simulink model "W04_Town_cs"  (R2019a)
settings: Solver=FixedStepDiscrete  StartTime=0.0  StopTime=15  FixedStep=1/20  RelTol=1e-3
PreLoadFcn:
  | mbxruntime.callbacks.PreLoadFcn(bdroot);
  | check_NUTS_defined
  | model_closed = 0;
  | assignin('base',['model_closed_' bdroot],false);
PostLoadFcn:
  | mbxruntime.callbacks.PostLoadFcn(bdroot);
InitFcn:
  | mbxruntime.callbacks.InitFcn(bdroot);
StartFcn:
  | mbxruntime.callbacks.StartFcn(bdroot);
StopFcn:
  | mbxruntime.callbacks.StopFcn(bdroot);;
  | 
model workspace: external: MAT-File .\W04_Town_cs_hws.mat (data not in the file)
undefined symbols (not defined in the file or in its folder): DiscIntNeverNeededParam, Header, InitImageOutputDir, Poses, Poses_SL_Info, W04_Town_cs_a800676c22972011, W04_Town_cs_bbf210301aa7dfc9, W04_Town_cs_BMW_X5_SUV_1_Dynamics_Empty_STATE_BMW_X5_SUV_1_x0, W04_Town_cs_BMW_X5_SUV_1_Dynamics_Empty_STATE_BMW_X5_SUV_1_y0, W04_Town_cs_BMW_X5_SUV_1_Dynamics_Empty_STATE_BMW_X5_SUV_1_Yaw0, W04_Town_cs_BMW_X5_SUV_1_Dynamics_Empty_STATE_BMW_X5_SUV_1_z0
libraries: adeye_lib x39, PreScanSimulinkLibrary x2, robotlib x2, PreScanUsefulBlocks x1
(part 2 of 3)

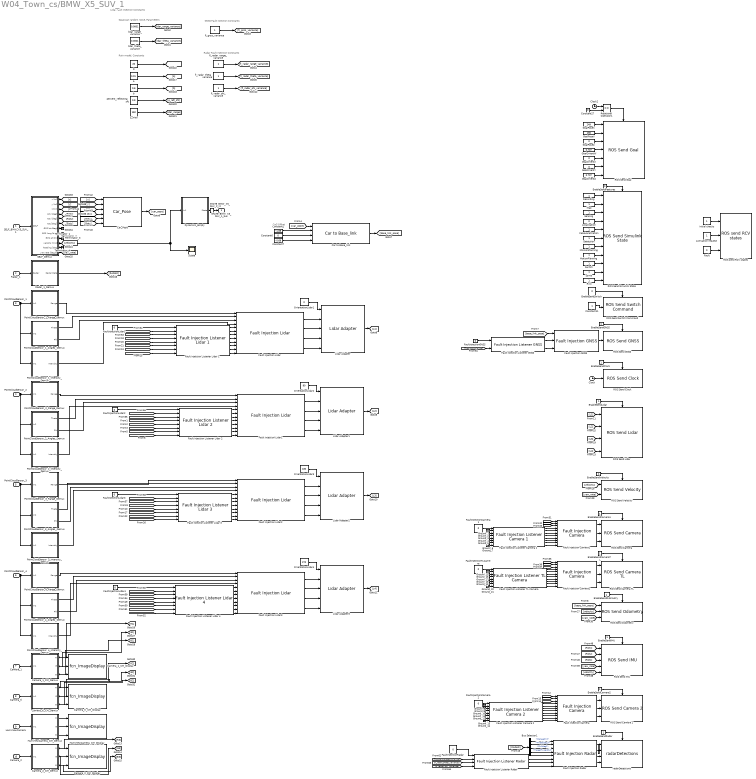
== system W04_Town_cs/BMW_X5_SUV_1 ==
  note: CoG Offset
  note: GNSS Fault Injection Constants
  note: Gaussian random noise, Parameters
  note: Radar Fault Injection Constants
  note: Lidar Fault injection Constants
  note: Rain model, Constants
  SELF_BMW_X5_SUV_1 : Inport  Tag=inport/SelfPort  OutDataTypeStr=Bus: PRESCAN_SELFSENSORDATA  PortDimensions=1  SampleTime=1/20  BusOutputAsStruct=on
  Radar_1 : Inport  Tag=inport/Radar  Port=2  OutDataTypeStr=Bus: PRESCAN_SCANNERSENSOR_MESSAGE  PortDimensions=7  SampleTime=1/20  BusOutputAsStruct=on
  PointCloudSensor_1 : Inport  Tag=inport/PointCloudInport  Port=3  OutDataTypeStr=single  SampleTime=1/20  BusOutputAsStruct=on
  PointCloudSensor_2 : Inport  Tag=inport/PointCloudInport  Port=4  OutDataTypeStr=single  SampleTime=1/20  BusOutputAsStruct=on
  PointCloudSensor_3 : Inport  Tag=inport/PointCloudInport  Port=5  OutDataTypeStr=single  SampleTime=1/20  BusOutputAsStruct=on
  PointCloudSensor_4 : Inport  Tag=inport/PointCloudInport  Port=6  OutDataTypeStr=single  SampleTime=1/20  BusOutputAsStruct=on
  Camera_1 : Inport  Tag=inport/Camera/CameraSensor  Port=7  OutDataTypeStr=uint8  SampleTime=1/20  BusOutputAsStruct=on
  Camera_tl : Inport  Tag=inport/Camera/CameraSensor  Port=8  OutDataTypeStr=uint8  SampleTime=1/20  BusOutputAsStruct=on
  HumViewCamera : Inport  Tag=inport/Camera/CameraSensor  Port=9  OutDataTypeStr=uint8  SampleTime=1/20  BusOutputAsStruct=on
  Camera_2 : Inport  Tag=inport/Camera/CameraSensor  Port=10  OutDataTypeStr=uint8  SampleTime=1/20  BusOutputAsStruct=on
  Activation request : Constant  OutDataTypeStr=Inherit: Inherit via back propagation
  Bus Selector1 : BusSelector  OutputSignals=Range[m],Theta[deg],Phi[deg],TargetTypeID[-]
  Camera_1_CM_Demux : Subsystem  Tag=demux/Camera/Color  mask{SensorName=Camera_1, hres=960, vres=720}
      mask prompts: SensorName "Sensor Name"; hres "Horizontal Resolution"; vres "Vertical Resolution"
      mask Help: eval('openHelp(457)')
      mask Display:
      | fprintf('MONO CAMERA:\n Color\n %s \n %d x %d px',SensorName,hres,vres)
      | port_label('output',1,'R')
      | port_label('output',2,'G')
      | port_label('output',3,'B')
  Camera_1_CM_Display : M-S-Function  Tag=CameraSensor_Color_Display  InitFcn=InitImageOutputDir(gcb);  FunctionName=fcn_ImageDisplay  Parameters=SensorName EnableDisplay EnablePosition DisplayPosition FigureHandle SaveResults BitmapFormat TempOutputDir CameraType DataType  mask(PreScan Color Display Block){SensorName=Camera_1, EnableDisplay=off, EnablePosition=off, DisplayPosition=[10 10 960 720], FigureHandle=1639205, SaveResults=off, Format=PNG, TempOutputDir=0, CameraType=Mono, DataType=uint8}
      mask prompts: SensorName "User Specified: Title of Display"; EnableDisplay "Active"; EnablePosition "Set Display window position"; DisplayPosition "Display window position [xpos ypos width height]"; FigureHandle "Unique Handle"; SaveResults "Save results"; TempOutputDir "OutputDir"; CameraType "Camera Type"; DataType "Image Data Type"
      mask help: This block displays the RGB output of a PreScan camera sensor.
      mask init:
      | if EnableDisplay
      |     EnableString='';
      |     EnableColor='gray';
      | else
      |     EnableString='INACTIVE';
      |     EnableColor='red';
      | end
      | switch Format
      |     case 1
      |         BitmapFormat = 'png';
      |     case 2
      |         BitmapFormat = 'bmp';
      |     case 3
      |         BitmapFormat = 'jpg';
      | end 
      | if CameraType==1
      |     CameraTypeName='MONO';
      |     PortNumber=0;
      | else
      |     CameraTypeName='STEREO';
      |     PortNumber=3;
      | end
      settings: CopyFcn=CopyFcnDisplay  DeleteFcn=PreScanBlockDeleteFcn;  ModelCloseFcn=fcn_ImageDisplay_ModelCloseFcn
      mask Help: eval('openHelp(457)')
      mask Callback EnablePosition:
      | MV=get_param(gcb,'MaskVisibilities');
      | if strcmp(get_param(gcb,'EnablePosition'),'on')
      |     MV{4}='on';
      | else
      |     MV{4}='off';
      | end
      | set_param(gcb,'MaskVisibilities',MV);
      | clear MV;
      mask TypeOptions Format: PNG | BMP | JPG
      mask TypeOptions CameraType: Mono | Stereo
      mask TypeOptions DataType: uint8 | single
      mask Display:
      | color(EnableColor);
      | fprintf('%s\n DISPLAY:\n Color \n %s',EnableString,SensorName)
      | port_label('input',1,'R')
      | port_label('input',2,'G')
      | port_label('input',3,'B')
      | port_label('input',PortNumber+1,'R')
      | port_label('input',PortNumber+2,'G')
      | port_label('input',PortNumber+3,'B')
  Camera_2_CM_Demux : Subsystem  Tag=demux/Camera/Color  mask{SensorName=Camera_2, hres=960, vres=720}
      mask prompts: SensorName "Sensor Name"; hres "Horizontal Resolution"; vres "Vertical Resolution"
      mask Help: eval('openHelp(457)')
      mask Display:
      | fprintf('MONO CAMERA:\n Color\n %s \n %d x %d px',SensorName,hres,vres)
      | port_label('output',1,'R')
      | port_label('output',2,'G')
      | port_label('output',3,'B')
  Camera_2_CM_Display : M-S-Function  Tag=CameraSensor_Color_Display  InitFcn=InitImageOutputDir(gcb);  FunctionName=fcn_ImageDisplay  Parameters=SensorName EnableDisplay EnablePosition DisplayPosition FigureHandle SaveResults BitmapFormat TempOutputDir CameraType DataType  mask(PreScan Color Display Block){SensorName=Camera_2, EnableDisplay=off, EnablePosition=off, DisplayPosition=[10 10 960 720], FigureHandle=1639208, SaveResults=off, Format=PNG, TempOutputDir=0, CameraType=Mono, DataType=uint8}
      mask prompts: SensorName "User Specified: Title of Display"; EnableDisplay "Active"; EnablePosition "Set Display window position"; DisplayPosition "Display window position [xpos ypos width height]"; FigureHandle "Unique Handle"; SaveResults "Save results"; TempOutputDir "OutputDir"; CameraType "Camera Type"; DataType "Image Data Type"
      mask help: This block displays the RGB output of a PreScan camera sensor.
      mask init: same as W04_Town_cs/BMW_X5_SUV_1/Camera_1_CM_Display
      settings: CopyFcn=CopyFcnDisplay  DeleteFcn=PreScanBlockDeleteFcn;  ModelCloseFcn=fcn_ImageDisplay_ModelCloseFcn
      mask Help: eval('openHelp(457)')
      mask Callback EnablePosition:
      | MV=get_param(gcb,'MaskVisibilities');
      | if strcmp(get_param(gcb,'EnablePosition'),'on')
      |     MV{4}='on';
      | else
      |     MV{4}='off';
      | end
      | set_param(gcb,'MaskVisibilities',MV);
      | clear MV;
      mask TypeOptions Format: PNG | BMP | JPG
      mask TypeOptions CameraType: Mono | Stereo
      mask TypeOptions DataType: uint8 | single
      mask Display:
      | color(EnableColor);
      | fprintf('%s\n DISPLAY:\n Color \n %s',EnableString,SensorName)
      | port_label('input',1,'R')
      | port_label('input',2,'G')
      | port_label('input',3,'B')
      | port_label('input',PortNumber+1,'R')
      | port_label('input',PortNumber+2,'G')
      | port_label('input',PortNumber+3,'B')
  Camera_tl_CM_Demux : Subsystem  Tag=demux/Camera/Color  mask{SensorName=Camera_tl, hres=960, vres=720}
      mask prompts: SensorName "Sensor Name"; hres "Horizontal Resolution"; vres "Vertical Resolution"
      mask Help: eval('openHelp(457)')
      mask Display:
      | fprintf('MONO CAMERA:\n Color\n %s \n %d x %d px',SensorName,hres,vres)
      | port_label('output',1,'R')
      | port_label('output',2,'G')
      | port_label('output',3,'B')
  Camera_tl_CM_Display : M-S-Function  Tag=CameraSensor_Color_Display  InitFcn=InitImageOutputDir(gcb);  FunctionName=fcn_ImageDisplay  Parameters=SensorName EnableDisplay EnablePosition DisplayPosition FigureHandle SaveResults BitmapFormat TempOutputDir CameraType DataType  mask(PreScan Color Display Block){SensorName=Camera_tl, EnableDisplay=off, EnablePosition=off, DisplayPosition=[10 10 960 720], FigureHandle=1639206, SaveResults=off, Format=PNG, TempOutputDir=0, CameraType=Mono, DataType=uint8}
      mask prompts: SensorName "User Specified: Title of Display"; EnableDisplay "Active"; EnablePosition "Set Display window position"; DisplayPosition "Display window position [xpos ypos width height]"; FigureHandle "Unique Handle"; SaveResults "Save results"; TempOutputDir "OutputDir"; CameraType "Camera Type"; DataType "Image Data Type"
      mask help: This block displays the RGB output of a PreScan camera sensor.
      mask init: same as W04_Town_cs/BMW_X5_SUV_1/Camera_1_CM_Display
      settings: CopyFcn=CopyFcnDisplay  DeleteFcn=PreScanBlockDeleteFcn;  ModelCloseFcn=fcn_ImageDisplay_ModelCloseFcn
      mask Help: eval('openHelp(457)')
      mask Callback EnablePosition:
      | MV=get_param(gcb,'MaskVisibilities');
      | if strcmp(get_param(gcb,'EnablePosition'),'on')
      |     MV{4}='on';
      | else
      |     MV{4}='off';
      | end
      | set_param(gcb,'MaskVisibilities',MV);
      | clear MV;
      mask TypeOptions Format: PNG | BMP | JPG
      mask TypeOptions CameraType: Mono | Stereo
      mask TypeOptions DataType: uint8 | single
      mask Display:
      | color(EnableColor);
      | fprintf('%s\n DISPLAY:\n Color \n %s',EnableString,SensorName)
      | port_label('input',1,'R')
      | port_label('input',2,'G')
      | port_label('input',3,'B')
      | port_label('input',PortNumber+1,'R')
      | port_label('input',PortNumber+2,'G')
      | port_label('input',PortNumber+3,'B')
  Car to Base_link : adeye_lib/Car to Base_link  SystemSampleTime=-1
  Car_Pose : adeye_lib/Car_Pose  SystemSampleTime=-1
  Clock : Clock
  Clock2 : Clock
  Constant11 : Constant  OutDataTypeStr=Inherit: Inherit via back propagation  SampleTime=0.05
  Constant2 : Constant  Value=-1.69
  Constant27 : Constant  Value=0
  Constant6 : Constant  Value=0
  Constant7 : Constant  Value=-0.69
  Detection : Constant
  Dynamics_Empty : Subsystem  Tag=Dynamics_Empty
      mask Help: eval('openHelp(202)')
      mask Display: port_label('output', 1, 'State');text(0,0,' Empty\n')
  EnableSendCamera1 : Constant  OutDataTypeStr=Inherit: Inherit via back propagation
  EnableSendCamera2 : Constant  OutDataTypeStr=Inherit: Inherit via back propagation
  EnableSendCameraTL : Constant  OutDataTypeStr=Inherit: Inherit via back propagation
  EnableSendClock : Constant  OutDataTypeStr=Inherit: Inherit via back propagation
  EnableSendFeatures : Constant  Value=0  OutDataTypeStr=Inherit: Inherit via back propagation
  EnableSendGNSS : Constant  OutDataTypeStr=Inherit: Inherit via back propagation
  EnableSendIMU : Constant  OutDataTypeStr=Inherit: Inherit via back propagation
  EnableSendLidar : Constant  OutDataTypeStr=Inherit: Inherit via back propagation
  EnableSendOdometry : Constant
  EnableSendRadar : Constant  OutDataTypeStr=Inherit: Inherit via back propagation
  EnableSendSwitch : Constant  Value=0  OutDataTypeStr=Inherit: Inherit via back propagation  SampleTime=0.05
  EnableSendVelocity : Constant  OutDataTypeStr=Inherit: Inherit via back propagation
  FakeLocalization : Constant
  Fault : Constant  Value=0  OutDataTypeStr=Inherit: Inherit via back propagation
  Fault Injection Camera : adeye_lib/Fault Injection Camera  idy=200  idx=100  x=100  y=150  R=0  G=0  B=0
  Fault Injection Camera1 : adeye_lib/Fault Injection Camera  idy=200  idx=100  x=100  y=150  R=0  G=0  B=0
  Fault Injection Camera2 : adeye_lib/Fault Injection Camera  idy=200  idx=100  x=100  y=150  R=0  G=0  B=0
  Fault Injection GNSS : adeye_lib/Fault Injection GNSS  f=20
  Fault Injection Lidar{,1..3} (4 alike) : adeye_lib/Fault Injection Lidar  f=20  p=225*16
  Fault Injection Listener Camera 1 : adeye_lib/Fault Injection Listener Camera 1  SystemSampleTime=-1
  Fault Injection Listener Camera 2 : adeye_lib/Fault Injection Listener Camera 2  SystemSampleTime=-1
  Fault Injection Listener GNSS : adeye_lib/Fault Injection Listener GNSS  SystemSampleTime=-1
  Fault Injection Listener Lidar 1 : adeye_lib/Fault Injection Listener Lidar 1  SystemSampleTime=-1
  Fault Injection Listener Lidar 2 : adeye_lib/Fault Injection Listener Lidar 2  SystemSampleTime=-1
  Fault Injection Listener Lidar 3 : adeye_lib/Fault Injection Listener Lidar 3  SystemSampleTime=-1
  Fault Injection Listener Lidar 4 : adeye_lib/Fault Injection Listener Lidar 4  SystemSampleTime=-1
  Fault Injection Listener Radar : adeye_lib/Fault Injection Listener Radar  SystemSampleTime=-1
  Fault Injection Listener TL Camera : adeye_lib/Fault Injection Listener TL Camera  SystemSampleTime=-1
  Fault Injection Radar : adeye_lib/Fault Injection Radar  n=7
  FaultInjectionCamera1 : Constant  Value=0
  FaultInjectionCamera2 : Constant  Value=0
  FaultInjectionGNSS : Constant  Value=0  OutDataTypeStr=Inherit: Inherit via back propagation  SampleTime=0.05
  FaultInjectionLidar{1..4} (4 alike) : Constant  Value=0  OutDataTypeStr=Inherit: Inherit via back propagation
  FaultInjectionRadar : Constant  Value=0
  FaultInjectionTLCamera : Constant  Value=0
  GoalOrientW : Constant  Value=0.707
  GoalOrientX : Constant  Value=0
  GoalOrientY : Constant  Value=0
  GoalOrientZ : Constant  Value=0.707
  GoalPoseX : Constant  Value=249
  GoalPoseY : Constant  Value=136
  GoalPoseZ : Constant  Value=0
  Ground_{1..21} (21 alike) : Ground
  HumViewCamera_CM_Demux : Subsystem  Tag=demux/Camera/Color  mask{SensorName=HumViewCamera, hres=1871, vres=1080}
      mask prompts: SensorName "Sensor Name"; hres "Horizontal Resolution"; vres "Vertical Resolution"
      mask Help: eval('openHelp(457)')
      mask Display:
      | fprintf('MONO CAMERA:\n Color\n %s \n %d x %d px',SensorName,hres,vres)
      | port_label('output',1,'R')
      | port_label('output',2,'G')
      | port_label('output',3,'B')
  HumViewCamera_CM_Display : M-S-Function  Tag=CameraSensor_Color_Display  InitFcn=InitImageOutputDir(gcb);  FunctionName=fcn_ImageDisplay  Parameters=SensorName EnableDisplay EnablePosition DisplayPosition FigureHandle SaveResults BitmapFormat TempOutputDir CameraType DataType  mask(PreScan Color Display Block){SensorName=HumViewCamera, EnableDisplay=off, EnablePosition=off, DisplayPosition=[10 10 1871 1080], FigureHandle=1639207, SaveResults=off, Format=PNG, TempOutputDir=0, CameraType=Mono, DataType=uint8}
      mask prompts: SensorName "User Specified: Title of Display"; EnableDisplay "Active"; EnablePosition "Set Display window position"; DisplayPosition "Display window position [xpos ypos width height]"; FigureHandle "Unique Handle"; SaveResults "Save results"; TempOutputDir "OutputDir"; CameraType "Camera Type"; DataType "Image Data Type"
      mask help: This block displays the RGB output of a PreScan camera sensor.
      mask init: same as W04_Town_cs/BMW_X5_SUV_1/Camera_1_CM_Display
      settings: CopyFcn=CopyFcnDisplay  DeleteFcn=PreScanBlockDeleteFcn;  ModelCloseFcn=fcn_ImageDisplay_ModelCloseFcn
      mask Help: eval('openHelp(457)')
      mask Callback EnablePosition:
      | MV=get_param(gcb,'MaskVisibilities');
      | if strcmp(get_param(gcb,'EnablePosition'),'on')
      |     MV{4}='on';
      | else
      |     MV{4}='off';
      | end
      | set_param(gcb,'MaskVisibilities',MV);
      | clear MV;
      mask TypeOptions Format: PNG | BMP | JPG
      mask TypeOptions CameraType: Mono | Stereo
      mask TypeOptions DataType: uint8 | single
      mask Display:
      | color(EnableColor);
      | fprintf('%s\n DISPLAY:\n Color \n %s',EnableString,SensorName)
      | port_label('input',1,'R')
      | port_label('input',2,'G')
      | port_label('input',3,'B')
      | port_label('input',PortNumber+1,'R')
      | port_label('input',PortNumber+2,'G')
      | port_label('input',PortNumber+3,'B')
  Initial checks : Constant  OutDataTypeStr=Inherit: Inherit via back propagation
  Lidar Adapter{,1..3} (4 alike) : adeye_lib/Lidar Adapter  SystemSampleTime=-1
  Localization : Constant  Value=0
  Map : Constant
  MissionPlanning : Constant
  MotionPlanning : Constant
  OrientationLidar1 : Constant  Value=0  OutDataTypeStr=Inherit: Inherit via back propagation
  OrientationLidar2 : Constant  Value=90  OutDataTypeStr=Inherit: Inherit via back propagation
  OrientationLidar3 : Constant  Value=180  OutDataTypeStr=Inherit: Inherit via back propagation
  OrientationLidar4 : Constant  Value=270  OutDataTypeStr=Inherit: Inherit via back propagation
  PointCloudSensor_1_Angles_Demux : Subsystem  Tag=demux/PCS/Angles  mask{SensorName=PointCloudSensor_1, offset=225, hres=225, vres=16}
      mask prompts: SensorName "Sensor Name"; offset "Data Start"; hres "Horizontal Resolution"; vres "Vertical Resolution"
      mask Help: eval('openHelp(6400)')
      mask Display:
      | fprintf('Point Cloud:\n Data\n %s \n %d x %d px',SensorName,hres,vres)
      | port_label('output',1,'Theta')
      | port_label('output',2,'Phi')
  PointCloudSensor_1_Intensity_Demux : Subsystem  Tag=demux/PCS/Intensity  mask{SensorName=PointCloudSensor_1, offset=675, hres=225, vres=16}
      mask prompts: SensorName "Sensor Name"; offset "Data Start"; hres "Horizontal Resolution"; vres "Vertical Resolution"
      mask Help: eval('openHelp(6400)')
      mask Display:
      | fprintf('Point Cloud:\n Data\n %s \n %d x %d px',SensorName,hres,vres)
      | port_label('output',1,'Intensity')
  PointCloudSensor_1_Range_Demux : Subsystem  Tag=demux/PCS/Range  mask{SensorName=PointCloudSensor_1, offset=0, hres=225, vres=16}
      mask prompts: SensorName "Sensor Name"; offset "Data Start"; hres "Horizontal Resolution"; vres "Vertical Resolution"
      mask Help: eval('openHelp(6400)')
      mask Display:
      | fprintf('Point Cloud:\n Data\n %s \n %d x %d px',SensorName,hres,vres)
      | port_label('output',1,'Range')
  PointCloudSensor_2_Angles_Demux : Subsystem  Tag=demux/PCS/Angles  mask{SensorName=PointCloudSensor_2, offset=225, hres=225, vres=16}
      mask prompts: SensorName "Sensor Name"; offset "Data Start"; hres "Horizontal Resolution"; vres "Vertical Resolution"
      mask Help: eval('openHelp(6400)')
      mask Display:
      | fprintf('Point Cloud:\n Data\n %s \n %d x %d px',SensorName,hres,vres)
      | port_label('output',1,'Theta')
      | port_label('output',2,'Phi')
  PointCloudSensor_2_Intensity_Demux : Subsystem  Tag=demux/PCS/Intensity  mask{SensorName=PointCloudSensor_2, offset=675, hres=225, vres=16}
      mask prompts: SensorName "Sensor Name"; offset "Data Start"; hres "Horizontal Resolution"; vres "Vertical Resolution"
      mask Help: eval('openHelp(6400)')
      mask Display:
      | fprintf('Point Cloud:\n Data\n %s \n %d x %d px',SensorName,hres,vres)
      | port_label('output',1,'Intensity')
  PointCloudSensor_2_Range_Demux : Subsystem  Tag=demux/PCS/Range  mask{SensorName=PointCloudSensor_2, offset=0, hres=225, vres=16}
      mask prompts: SensorName "Sensor Name"; offset "Data Start"; hres "Horizontal Resolution"; vres "Vertical Resolution"
      mask Help: eval('openHelp(6400)')
      mask Display:
      | fprintf('Point Cloud:\n Data\n %s \n %d x %d px',SensorName,hres,vres)
      | port_label('output',1,'Range')
  PointCloudSensor_3_Angles_Demux : Subsystem  Tag=demux/PCS/Angles  mask{SensorName=PointCloudSensor_3, offset=225, hres=225, vres=16}
      mask prompts: SensorName "Sensor Name"; offset "Data Start"; hres "Horizontal Resolution"; vres "Vertical Resolution"
      mask Help: eval('openHelp(6400)')
      mask Display:
      | fprintf('Point Cloud:\n Data\n %s \n %d x %d px',SensorName,hres,vres)
      | port_label('output',1,'Theta')
      | port_label('output',2,'Phi')
  PointCloudSensor_3_Intensity_Demux : Subsystem  Tag=demux/PCS/Intensity  mask{SensorName=PointCloudSensor_3, offset=675, hres=225, vres=16}
      mask prompts: SensorName "Sensor Name"; offset "Data Start"; hres "Horizontal Resolution"; vres "Vertical Resolution"
      mask Help: eval('openHelp(6400)')
      mask Display:
      | fprintf('Point Cloud:\n Data\n %s \n %d x %d px',SensorName,hres,vres)
      | port_label('output',1,'Intensity')
  PointCloudSensor_3_Range_Demux : Subsystem  Tag=demux/PCS/Range  mask{SensorName=PointCloudSensor_3, offset=0, hres=225, vres=16}
      mask prompts: SensorName "Sensor Name"; offset "Data Start"; hres "Horizontal Resolution"; vres "Vertical Resolution"
      mask Help: eval('openHelp(6400)')
      mask Display:
      | fprintf('Point Cloud:\n Data\n %s \n %d x %d px',SensorName,hres,vres)
      | port_label('output',1,'Range')
  PointCloudSensor_4_Angles_Demux : Subsystem  Tag=demux/PCS/Angles  mask{SensorName=PointCloudSensor_4, offset=225, hres=225, vres=16}
      mask prompts: SensorName "Sensor Name"; offset "Data Start"; hres "Horizontal Resolution"; vres "Vertical Resolution"
      mask Help: eval('openHelp(6400)')
      mask Display:
      | fprintf('Point Cloud:\n Data\n %s \n %d x %d px',SensorName,hres,vres)
      | port_label('output',1,'Theta')
      | port_label('output',2,'Phi')
  PointCloudSensor_4_Intensity_Demux : Subsystem  Tag=demux/PCS/Intensity  mask{SensorName=PointCloudSensor_4, offset=675, hres=225, vres=16}
      mask prompts: SensorName "Sensor Name"; offset "Data Start"; hres "Horizontal Resolution"; vres "Vertical Resolution"
      mask Help: eval('openHelp(6400)')
      mask Display:
      | fprintf('Point Cloud:\n Data\n %s \n %d x %d px',SensorName,hres,vres)
      | port_label('output',1,'Intensity')
  PointCloudSensor_4_Range_Demux : Subsystem  Tag=demux/PCS/Range  mask{SensorName=PointCloudSensor_4, offset=0, hres=225, vres=16}
      mask prompts: SensorName "Sensor Name"; offset "Data Start"; hres "Horizontal Resolution"; vres "Vertical Resolution"
      mask Help: eval('openHelp(6400)')
      mask Display:
      | fprintf('Point Cloud:\n Data\n %s \n %d x %d px',SensorName,hres,vres)
      | port_label('output',1,'Range')
  R : Constant  Value=20
  ROS Send Camera : adeye_lib/ROS Send Camera  SystemSampleTime=-1
  ROS Send Camera 2 : adeye_lib/ROS Send Camera 2  SystemSampleTime=-1
  ROS Send Camera TL : adeye_lib/ROS Send Camera TL  SystemSampleTime=-1
  ROS Send Clock : adeye_lib/ROS Send Clock  SystemSampleTime=-1
  ROS Send GNSS : adeye_lib/ROS Send GNSS  SystemSampleTime=-1
  ROS Send Goal : adeye_lib/ROS Send Goal  SystemSampleTime=-1
  ROS Send IMU : adeye_lib/ROS Send IMU  SystemSampleTime=-1
  ROS Send Lidar : adeye_lib/ROS Send Lidar  SystemSampleTime=-1
  ROS Send Odometry : adeye_lib/ROS Send Odometry  SystemSampleTime=-1
  ROS Send Simulink State : adeye_lib/ROS Send Simulink State  SystemSampleTime=-1
  ROS Send Switch Command : adeye_lib/ROS Send Switch Command  SystemSampleTime=-1
  ROS Send Velocity : adeye_lib/ROS Send Velocity  SystemSampleTime=-1
  ROS send RCV states : adeye_lib/ROS send RCV states  SystemSampleTime=-1
  Radar_1_Demux : Subsystem  Tag=demux/Radar  TreatAsAtomicUnit=on  mask(PreScan Demux Block: Radar){MAXMESSAGES=7}
      mask prompts: MAXMESSAGES "Number of Objects"
      mask help:
      | The Radar Sensor is a detailed sensor based on a physical radar
      | model that includes Antenna GAIN Maps (AGM) and atmospheric
      | attenuation.
      |
      | For more information, please click Help.
      mask Help: eval('openHelp(1464)')
      mask Display:
      | port_label('input',1,'Radar')
      | port_label('output',1,'Radar Data')
  Recording : Constant
  Relational Operator1 : RelationalOperator  Operator===  OutDataTypeStr=boolean  RndMeth=Simplest
  Rviz : Constant
  SELF_Demux : Subsystem  Tag=demux/SelfPort  mask(PreScan Demux Block:){}
      mask help:
      | The SELF port shows (state) information of the actor itself. The outputs are position in the experiment's axis system and the GPS coordinates, and the object's absolute velocity and compass heading.
      |
      | For more information, please click Help.
      settings: DeleteFcn=PreScanBlockDeleteFcn;
      mask Help: eval('openHelp(462)')
      mask Display:
      | port_label('output',1,'x [m]')
      | port_label('output',2,'y [m]')
      | port_label('output',3,'z [m]','texmode','on')
      | port_label('output',4,'Rotx [deg]','texmode','on')
      | port_label('output',5,'Roty [deg]','texmode','on')
      | port_label('output',6,'Rotz [deg]','texmode','on')
      | port_label('output',7,'GPS lat [deg]','texmode','on')
      | port_label('output',8,'GPS long [deg]','texmode','on')
      | port_label('output',9,'GPS alt [m]','texmode','on')
      | port_label('output',10,'Velocity [m/s]')
      | port_label('output',11,'Heading [deg]')
      | port_label('output',12,'Yaw rate [deg/s]')
  STATE_BMW_X5_SUV_1_rc : RateTransition  Tag=mux_rc/StatePort  OutPortSampleTimeOpt=Inherit
  Scope : Scope
  Sensing : Constant
  Ssmp : Constant
  Switch : Constant
  Terminator_{1..4} (4 alike) : Terminator
  a : Constant  Value=0.01
  b : Constant  Value=0.6
  fi_gnss_variance : Constant
  fi_radar_phi_variance : Constant
  fi_radar_range_variance : Constant
  fi_radar_theta_variance : Constant
  lidar_range_variance : Constant  Value=0.0001
  lidar_theta_variance : Constant  Value=0.0001
  percent_reflecting_sfc : Constant  Value=0.9
  radarDetections : adeye_lib/radarDetections  SystemSampleTime=-1
  z_max : Constant  Value=150
  STATE_BMW_X5_SUV_1_bus : Outport  Tag=outport/StatePort  OutDataTypeStr=Bus: PRESCAN_STATEACTUATORDATA  PortDimensions=1  SampleTime=1/20
  wires:
  [x] -> Car_Pose/1
  [y] -> Car_Pose/2
  [z] -> Car_Pose/3
  [Rotx] -> Car_Pose/4
  [Roty] -> Car_Pose/5
  [Rotz] -> Car_Pose/6
  SELF_Demux/12(yaw rate [deg/s]) -> [yaw_rate]
  SELF_Demux/1(x [m]) -> [x]
  SELF_Demux/6(rotz [deg]) -> [Rotz]
  SELF_Demux/5(roty [deg]) -> [Roty]
  SELF_Demux/4(rotx [deg]) -> [Rotx]
  SELF_Demux/3(z [m]) -> [z]
  SELF_Demux/2(y [m]) -> [y]
  Camera_1_CM_Demux/1(R) -> [R1], Camera_1_CM_Display/1
  Camera_1_CM_Demux/2(G) -> [G1], Camera_1_CM_Display/2
  Camera_1_CM_Demux/3(B) -> [B1], Camera_1_CM_Display/3
  Camera_tl_CM_Demux/1(R) -> [R2], Camera_tl_CM_Display/1
  Camera_tl_CM_Demux/2(G) -> [G2], Camera_tl_CM_Display/2
  Camera_tl_CM_Demux/3(B) -> [B2], Camera_tl_CM_Display/3
  Camera_2_CM_Demux/1(R) -> [R3], Camera_2_CM_Display/1
  Camera_2_CM_Demux/2(G) -> [G3], Camera_2_CM_Display/2
  Camera_2_CM_Demux/3(B) -> [B3], Camera_2_CM_Display/3
  Car_Pose/1 -> [car_pose]
  SELF_Demux/10(velocity [m/s]) -> Scope/1, Dynamics_Empty/1(In1), [velocity]
  Radar_1_Demux/1(Radar Data) -> [RADAR]
  [car_pose] -> Car to Base_link/1
  Constant7/1 -> Car to Base_link/4
  Constant6/1 -> Car to Base_link/3
  Car to Base_link/1 -> [base_link_pose]
  Constant2/1 -> Car to Base_link/2
  Fault Injection Camera2/3 -> ROS Send Camera TL/3
  Ssmp/1 -> ROS Send Simulink State/10
  Fault Injection Listener TL Camera/7 -> Fault Injection Camera2/10
  [fi_radar_phi_variance] -> Fault Injection Listener Radar/4
  [G2] -> Fault Injection Camera2/2
  [fi_radar_theta_variance] -> Fault Injection Listener Radar/3
  [fi_radar_range_variance] -> Fault Injection Listener Radar/2
  Fault Injection Listener Camera 2/3 -> Fault Injection Camera/6
  GoalOrientZ/1 -> ROS Send Goal/7
  Fault Injection Listener Camera 1/4 -> Fault Injection Camera1/7
  EnableSendFeatures/1 -> ROS Send Simulink State/Enable
  Fault Injection Listener Radar/4 -> Fault Injection Radar/8
  Fault Injection Listener Radar/3 -> Fault Injection Radar/7
  EnableSendGNSS/1 -> ROS Send GNSS/Enable
  Fault Injection Listener Camera 2/7 -> Fault Injection Camera/10
  Fault Injection Listener Camera 2/4 -> Fault Injection Camera/7
  [yaw_rate] -> ROS Send IMU/4
  Fault/1 -> ROS send RCV states/3
  Fault Injection Listener Camera 2/8 -> Fault Injection Camera/11
  Fault Injection Listener Camera 2/5 -> Fault Injection Camera/8
  Fault Injection Listener Camera 1/7 -> Fault Injection Camera1/10
  Fault Injection Radar/2 -> radarDetections/2
  Fault Injection Listener Camera 1/3 -> Fault Injection Camera1/6
  GoalOrientW/1 -> ROS Send Goal/4
  [G1] -> Fault Injection Camera1/2
  EnableSendSwitch/1 -> ROS Send Switch Command/Enable
  Fault Injection Listener TL Camera/6 -> Fault Injection Camera2/9
  Fault Injection Listener Camera 1/6 -> Fault Injection Camera1/9
  Fault Injection Listener TL Camera/2 -> Fault Injection Camera2/5
  [fi_gnss_variance] -> Fault Injection Listener GNSS/2
  Fault Injection Listener Camera 1/2 -> Fault Injection Camera1/5
  Fault Injection Listener Camera 1/8 -> Fault Injection Camera1/11
  MissionPlanning/1 -> ROS Send Simulink State/7
  Fault Injection Listener TL Camera/5 -> Fault Injection Camera2/8
  Fault Injection Listener TL Camera/3 -> Fault Injection Camera2/6
  Fault Injection Listener TL Camera/4 -> Fault Injection Camera2/7
  Detection/1 -> ROS Send Simulink State/6
  Fault Injection Listener Camera 2/2 -> Fault Injection Camera/5
  GoalOrientX/1 -> ROS Send Goal/5
  Fault Injection Listener Camera 2/6 -> Fault Injection Camera/9
  [L4] -> ROS Send Lidar/4
  GoalOrientY/1 -> ROS Send Goal/6
  EnableSendLidar/1 -> ROS Send Lidar/Enable
  Fault Injection GNSS/1 -> ROS Send GNSS/1
  [velocity] -> ROS Send Odometry/2
  Fault Injection Camera1/3 -> ROS Send Camera/3
  Fault Injection Camera1/2 -> ROS Send Camera/2
  Recording/1 -> ROS Send Simulink State/1
  EnableSendClock/1 -> ROS Send Clock/Enable
  Fault Injection Camera/3 -> ROS Send Camera 2/3
  [L1] -> ROS Send Lidar/1
  Bus Selector1/1 -> Fault Injection Radar/1  "<Range[m]>"
  EnableSendIMU/1 -> ROS Send IMU/Enable
  Fault Injection Listener Camera 1/1 -> Fault Injection Camera1/4
  [base_link_pose] -> Fault Injection GNSS/1
  Fault Injection Listener Camera 2/1 -> Fault Injection Camera/4
  FaultInjectionRadar/1 -> Fault Injection Listener Radar/1
  Fault Injection Camera2/2 -> ROS Send Camera TL/2
  FaultInjectionCamera2/1 -> Fault Injection Listener Camera 2/1
  [R3] -> Fault Injection Camera/1
  [G3] -> Fault Injection Camera/2
  Fault Injection Camera2/1 -> ROS Send Camera TL/1
  [B3] -> Fault Injection Camera/3
  Activation request/1 -> ROS send RCV states/2
  [B1] -> Fault Injection Camera1/3
  [R2] -> Fault Injection Camera2/1
  [L3] -> ROS Send Lidar/3
  [Roty] -> ROS Send IMU/2
  Initial checks/1 -> ROS send RCV states/1
  Fault Injection Listener Radar/1 -> Fault Injection Radar/5
  Fault Injection Radar/4 -> radarDetections/4
  Fault Injection Listener GNSS/1 -> Fault Injection GNSS/2
  GoalPoseX/1 -> ROS Send Goal/1
  Fault Injection Listener Radar/2 -> Fault Injection Radar/6
  FakeLocalization/1 -> ROS Send Simulink State/5
  GoalPoseY/1 -> ROS Send Goal/2
  GoalPoseZ/1 -> ROS Send Goal/3
  FaultInjectionCamera1/1 -> Fault Injection Listener Camera 1/1
  FaultInjectionTLCamera/1 -> Fault Injection Listener TL Camera/1
  Switch/1 -> ROS Send Simulink State/9
  EnableSendCamera2/1 -> ROS Send Camera 2/Enable
  Fault Injection Listener Camera 1/5 -> Fault Injection Camera1/8
  Localization/1 -> ROS Send Simulink State/4
  [yaw_rate] -> ROS Send Velocity/2
  FaultInjectionGNSS/1 -> Fault Injection Listener GNSS/1
  EnableSendCamera1/1 -> ROS Send Camera/Enable
  EnableSendCameraTL/1 -> ROS Send Camera TL/Enable
  [velocity] -> ROS Send IMU/5
  [Rotz] -> ROS Send IMU/3
  Fault Injection Camera1/1 -> ROS Send Camera/1
  EnableSendVelocity/1 -> ROS Send Velocity/Enable
  Fault Injection Camera/1 -> ROS Send Camera 2/1
  Constant27/1 -> Relational Operator1/2
  [yaw_rate] -> ROS Send Odometry/3
  [velocity] -> ROS Send Velocity/1
  [L2] -> ROS Send Lidar/2
  Fault Injection Listener TL Camera/8 -> Fault Injection Camera2/11
  Map/1 -> ROS Send Simulink State/2
  Sensing/1 -> ROS Send Simulink State/3
  [R1] -> Fault Injection Camera1/1
  [base_link_pose] -> ROS Send Odometry/1
  [Rotx] -> ROS Send IMU/1
  Relational Operator1/1 -> ROS Send Goal/Enable
  EnableSendOdometry/1 -> ROS Send Odometry/Enable
  Clock2/1 -> Relational Operator1/1
  Constant11/1 -> ROS Send Switch Command/1
  [B2] -> Fault Injection Camera2/3
  [RADAR] -> Bus Selector1/1
  Fault Injection Camera/2 -> ROS Send Camera 2/2
  Bus Selector1/3 -> Fault Injection Radar/3  "<Phi[deg]>"
  Fault Injection Radar/3 -> radarDetections/3
  Fault Injection Listener TL Camera/1 -> Fault Injection Camera2/4
  Bus Selector1/2 -> Fault Injection Radar/2  "<Theta[deg]>"
  EnableSendRadar/1 -> radarDetections/Enable
  Rviz/1 -> ROS Send Simulink State/11
  Clock/1 -> ROS Send Clock/1
  Fault Injection Radar/1 -> radarDetections/1
  Fault Injection Listener GNSS/2 -> Fault Injection GNSS/3
  Bus Selector1/4 -> Fault Injection Radar/4  "<TargetTypeID[-]>"
  MotionPlanning/1 -> ROS Send Simulink State/8
  [rain_intensity] -> Fault Injection Listener Lidar 4/4
  [lidar_range_variance] -> Fault Injection Listener Lidar 1/2
  [b] -> Fault Injection Listener Lidar 3/6
  [p_refl_sfc] -> Fault Injection Listener Lidar 2/7
  Fault Injection Lidar2/3 -> Lidar Adapter2/4
  [p_refl_sfc] -> Fault Injection Listener Lidar 3/7
  Fault Injection Listener Lidar 2/4 -> Fault Injection Lidar1/8
  [lidar_range] -> Fault Injection Listener Lidar 1/8
  [a] -> Fault Injection Listener Lidar 4/5
  [lidar_range] -> Fault Injection Listener Lidar 4/8
  Fault Injection Listener Lidar 2/5 -> Fault Injection Lidar1/9
  Fault Injection Lidar2/2 -> Lidar Adapter2/3
  [rain_intensity] -> Fault Injection Listener Lidar 3/4
  [rain_intensity] -> Fault Injection Listener Lidar 1/4
  [lidar_theta_variance] -> Fault Injection Listener Lidar 4/3
  [b] -> Fault Injection Listener Lidar 4/6
  Fault Injection Listener Lidar 3/6 -> Fault Injection Lidar2/10
  Lidar Adapter2/1 -> [L3]
  Lidar Adapter3/1 -> [L4]
  Fault Injection Listener Lidar 4/6 -> Fault Injection Lidar3/10
  Fault Injection Lidar3/3 -> Lidar Adapter3/4
  Fault Injection Listener Lidar 2/8 -> Fault Injection Lidar1/12
  Fault Injection Listener Lidar 3/2 -> Fault Injection Lidar2/6
  [a] -> Fault Injection Listener Lidar 3/5
  PointCloudSensor_2_Intensity_Demux/1(Intensity) -> Fault Injection Lidar1/4
  [b] -> Fault Injection Listener Lidar 2/6
  [lidar_range] -> Fault Injection Listener Lidar 2/8
  [lidar_theta_variance] -> Fault Injection Listener Lidar 3/3
  Fault Injection Listener Lidar 1/1 -> Fault Injection Lidar/5
  Fault Injection Listener Lidar 4/5 -> Fault Injection Lidar3/9
  [lidar_range_variance] -> Fault Injection Listener Lidar 4/2
  [lidar_range] -> Fault Injection Listener Lidar 3/8
  [lidar_theta_variance] -> Fault Injection Listener Lidar 2/3
  Fault Injection Listener Lidar 3/4 -> Fault Injection Lidar2/8
  [a] -> Fault Injection Listener Lidar 2/5
  Lidar Adapter/1 -> [L1]
  [lidar_range_variance] -> Fault Injection Listener Lidar 3/2
  Fault Injection Lidar3/1 -> Lidar Adapter3/2
  [rain_intensity] -> Fault Injection Listener Lidar 2/4
  Fault Injection Listener Lidar 1/2 -> Fault Injection Lidar/6
  PointCloudSensor_1_Range_Demux/1(Range) -> Fault Injection Lidar/1
  Fault Injection Listener Lidar 1/8 -> Fault Injection Lidar/12
  [p_refl_sfc] -> Fault Injection Listener Lidar 4/7
  PointCloudSensor_1_Angles_Demux/2(Phi) -> Fault Injection Lidar/3
  FaultInjectionLidar3/1 -> Fault Injection Listener Lidar 3/1
  [lidar_theta_variance] -> Fault Injection Listener Lidar 1/3
  Fault Injection Listener Lidar 4/7 -> Fault Injection Lidar3/11
  Fault Injection Listener Lidar 4/1 -> Fault Injection Lidar3/5
  Fault Injection Listener Lidar 4/4 -> Fault Injection Lidar3/8
  Fault Injection Listener Lidar 1/5 -> Fault Injection Lidar/9
  Fault Injection Listener Lidar 1/6 -> Fault Injection Lidar/10
  Fault Injection Lidar2/4 -> Lidar Adapter2/5
  PointCloudSensor_3_Range_Demux/1(Range) -> Fault Injection Lidar2/1
  Fault Injection Listener Lidar 1/7 -> Fault Injection Lidar/11
  Fault Injection Listener Lidar 3/1 -> Fault Injection Lidar2/5
  Fault Injection Listener Lidar 3/3 -> Fault Injection Lidar2/7
  Fault Injection Lidar1/3 -> Lidar Adapter1/4
  Fault Injection Listener Lidar 4/2 -> Fault Injection Lidar3/6
  PointCloudSensor_3_Angles_Demux/1(Theta) -> Fault Injection Lidar2/2
  Fault Injection Listener Lidar 3/5 -> Fault Injection Lidar2/9
  PointCloudSensor_3_Angles_Demux/2(Phi) -> Fault Injection Lidar2/3
  Fault Injection Lidar1/2 -> Lidar Adapter1/3
  Fault Injection Listener Lidar 1/4 -> Fault Injection Lidar/8
  Fault Injection Listener Lidar 2/3 -> Fault Injection Lidar1/7
  Fault Injection Lidar1/4 -> Lidar Adapter1/5
  Fault Injection Listener Lidar 2/7 -> Fault Injection Lidar1/11
  Fault Injection Listener Lidar 2/1 -> Fault Injection Lidar1/5
  OrientationLidar4/1 -> Lidar Adapter3/1
  Fault Injection Lidar1/1 -> Lidar Adapter1/2
  Fault Injection Listener Lidar 2/2 -> Fault Injection Lidar1/6
  [a] -> Fault Injection Listener Lidar 1/5
  Fault Injection Listener Lidar 1/3 -> Fault Injection Lidar/7
  [p_refl_sfc] -> Fault Injection Listener Lidar 1/7
  [b] -> Fault Injection Listener Lidar 1/6
  Fault Injection Lidar/1 -> Lidar Adapter/2
  Fault Injection Listener Lidar 3/7 -> Fault Injection Lidar2/11
  FaultInjectionLidar1/1 -> Fault Injection Listener Lidar 1/1
  FaultInjectionLidar4/1 -> Fault Injection Listener Lidar 4/1
  FaultInjectionLidar2/1 -> Fault Injection Listener Lidar 2/1
  Fault Injection Lidar2/1 -> Lidar Adapter2/2
  Fault Injection Listener Lidar 2/6 -> Fault Injection Lidar1/10
  [lidar_range_variance] -> Fault Injection Listener Lidar 2/2
  Fault Injection Lidar/2 -> Lidar Adapter/3
  PointCloudSensor_4_Angles_Demux/2(Phi) -> Fault Injection Lidar3/3
  PointCloudSensor_3_Intensity_Demux/1(Intensity) -> Fault Injection Lidar2/4
  Fault Injection Listener Lidar 4/3 -> Fault Injection Lidar3/7
  Fault Injection Lidar/3 -> Lidar Adapter/4
  Fault Injection Listener Lidar 3/8 -> Fault Injection Lidar2/12
  Fault Injection Lidar/4 -> Lidar Adapter/5
  Lidar Adapter1/1 -> [L2]
  OrientationLidar3/1 -> Lidar Adapter2/1
  PointCloudSensor_2_Range_Demux/1(Range) -> Fault Injection Lidar1/1
  Fault Injection Lidar3/4 -> Lidar Adapter3/5
  PointCloudSensor_1_Intensity_Demux/1(Intensity) -> Fault Injection Lidar/4
  Fault Injection Listener Lidar 4/8 -> Fault Injection Lidar3/12
  Fault Injection Lidar3/2 -> Lidar Adapter3/3
  OrientationLidar2/1 -> Lidar Adapter1/1
  PointCloudSensor_4_Angles_Demux/1(Theta) -> Fault Injection Lidar3/2
  PointCloudSensor_4_Range_Demux/1(Range) -> Fault Injection Lidar3/1
  PointCloudSensor_4_Intensity_Demux/1(Intensity) -> Fault Injection Lidar3/4
  PointCloudSensor_1_Angles_Demux/1(Theta) -> Fault Injection Lidar/2
  PointCloudSensor_2_Angles_Demux/1(Theta) -> Fault Injection Lidar1/2
  PointCloudSensor_2_Angles_Demux/2(Phi) -> Fault Injection Lidar1/3
  OrientationLidar1/1 -> Lidar Adapter/1
  fi_radar_phi_variance/1 -> [fi_radar_phi_variance]
  fi_gnss_variance/1 -> [fi_gnss_variance]
  lidar_range_variance/1 -> [lidar_range_variance]
  z_max/1 -> [lidar_range]
  percent_reflecting_sfc/1 -> [p_refl_sfc]
  R/1 -> [rain_intensity]
  b/1 -> [b]
  fi_radar_range_variance/1 -> [fi_radar_range_variance]
  fi_radar_theta_variance/1 -> [fi_radar_theta_variance]
  lidar_theta_variance/1 -> [lidar_theta_variance]
  a/1 -> [a]
  STATE_BMW_X5_SUV_1_rc/1 -> STATE_BMW_X5_SUV_1_bus/1
  SELF_BMW_X5_SUV_1/1 -> SELF_Demux/1(SELF)
  Radar_1/1 -> Radar_1_Demux/1(Radar)
  PointCloudSensor_1/1 -> PointCloudSensor_1_Range_Demux/1(In1), PointCloudSensor_1_Angles_Demux/1(In2), PointCloudSensor_1_Intensity_Demux/1(In1)
  PointCloudSensor_2/1 -> PointCloudSensor_2_Range_Demux/1(In1), PointCloudSensor_2_Angles_Demux/1(In2), PointCloudSensor_2_Intensity_Demux/1(In1)
  PointCloudSensor_3/1 -> PointCloudSensor_3_Range_Demux/1(In1), PointCloudSensor_3_Angles_Demux/1(In2), PointCloudSensor_3_Intensity_Demux/1(In1)
  PointCloudSensor_4/1 -> PointCloudSensor_4_Range_Demux/1(In1), PointCloudSensor_4_Angles_Demux/1(In2), PointCloudSensor_4_Intensity_Demux/1(In1)
  Camera_1/1 -> Camera_1_CM_Demux/1(In1)
  Camera_tl/1 -> Camera_tl_CM_Demux/1(In1)
  HumViewCamera/1 -> HumViewCamera_CM_Demux/1(In1)
  HumViewCamera_CM_Demux/1(R) -> HumViewCamera_CM_Display/1
  HumViewCamera_CM_Demux/2(G) -> HumViewCamera_CM_Display/2
  HumViewCamera_CM_Demux/3(B) -> HumViewCamera_CM_Display/3
  Camera_2/1 -> Camera_2_CM_Demux/1(In1)
  Dynamics_Empty/1(State) -> STATE_BMW_X5_SUV_1_rc/1
  Ground_1/1 -> Fault Injection Listener Camera 1/2
  Ground_2/1 -> Fault Injection Listener Camera 1/3
  Ground_3/1 -> Fault Injection Listener Camera 1/4
  Ground_4/1 -> Fault Injection Listener Camera 1/5
  Ground_5/1 -> Fault Injection Listener Camera 1/6
  Ground_6/1 -> Fault Injection Listener Camera 1/7
  Ground_7/1 -> Fault Injection Listener Camera 1/8
  Ground_8/1 -> Fault Injection Listener Camera 2/2
  Ground_9/1 -> Fault Injection Listener Camera 2/3
  Ground_10/1 -> Fault Injection Listener Camera 2/4
  Ground_11/1 -> Fault Injection Listener Camera 2/5
  Ground_12/1 -> Fault Injection Listener Camera 2/6
  Ground_13/1 -> Fault Injection Listener Camera 2/7
  Ground_14/1 -> Fault Injection Listener Camera 2/8
  Ground_15/1 -> Fault Injection Listener TL Camera/2
  Ground_16/1 -> Fault Injection Listener TL Camera/3
  Ground_17/1 -> Fault Injection Listener TL Camera/4
  Ground_18/1 -> Fault Injection Listener TL Camera/5
  Ground_19/1 -> Fault Injection Listener TL Camera/6
  Ground_20/1 -> Fault Injection Listener TL Camera/7
  Ground_21/1 -> Fault Injection Listener TL Camera/8
  SELF_Demux/7(GPS lat [deg]) -> Terminator_1/1
  SELF_Demux/8(GPS long [deg]) -> Terminator_2/1
  SELF_Demux/9(GPS alt [m]) -> Terminator_3/1
  SELF_Demux/11(heading [deg]) -> Terminator_4/1

== system W04_Town_cs/Camera_1 ==
  Sensor : S-Function  FunctionName=sfun_Camera  Parameters=sensorID, dataWidth, dataHeight, channelsPerImage, numberOfImages, timestep  SFunctionDeploymentMode=off  EnableBusSupport=off  mask(PreScan Source Block: Camera Sensor){sensorID=16397, dataWidth=720, dataHeight=2880, channelsPerImage=3, numberOfImages=1, timestep=1/20}
      mask prompts: sensorID "Sensor ID"; dataWidth "Data width"; dataHeight "Data Height"; channelsPerImage "Channels per image"; numberOfImages "Number of images"; timestep "MATLAB timestep:"
      mask help: The Camera Sensor provides a color or monochrome image.
      mask Help: eval('openHelp(457)')
      mask Display: image(imread('CameraSensor.png'))
  Camera_1 : Outport  Tag=outport/Camera/CameraSensor  OutDataTypeStr=uint8  SampleTime=1/20
  wires:
  Sensor/1 -> Camera_1/1

== system W04_Town_cs/Camera_2 ==
  Sensor : S-Function  FunctionName=sfun_Camera  Parameters=sensorID, dataWidth, dataHeight, channelsPerImage, numberOfImages, timestep  SFunctionDeploymentMode=off  EnableBusSupport=off  mask(PreScan Source Block: Camera Sensor){sensorID=16401, dataWidth=720, dataHeight=2880, channelsPerImage=3, numberOfImages=1, timestep=1/20}
      mask prompts: sensorID "Sensor ID"; dataWidth "Data width"; dataHeight "Data Height"; channelsPerImage "Channels per image"; numberOfImages "Number of images"; timestep "MATLAB timestep:"
      mask help: The Camera Sensor provides a color or monochrome image.
      mask Help: eval('openHelp(457)')
      mask Display: image(imread('CameraSensor.png'))
  Camera_2 : Outport  Tag=outport/Camera/CameraSensor  OutDataTypeStr=uint8  SampleTime=1/20
  wires:
  Sensor/1 -> Camera_2/1

== system W04_Town_cs/Camera_tl ==
  Sensor : S-Function  FunctionName=sfun_Camera  Parameters=sensorID, dataWidth, dataHeight, channelsPerImage, numberOfImages, timestep  SFunctionDeploymentMode=off  EnableBusSupport=off  mask(PreScan Source Block: Camera Sensor){sensorID=16398, dataWidth=720, dataHeight=2880, channelsPerImage=3, numberOfImages=1, timestep=1/20}
      mask prompts: sensorID "Sensor ID"; dataWidth "Data width"; dataHeight "Data Height"; channelsPerImage "Channels per image"; numberOfImages "Number of images"; timestep "MATLAB timestep:"
      mask help: The Camera Sensor provides a color or monochrome image.
      mask Help: eval('openHelp(457)')
      mask Display: image(imread('CameraSensor.png'))
  Camera_tl : Outport  Tag=outport/Camera/CameraSensor  OutDataTypeStr=uint8  SampleTime=1/20
  wires:
  Sensor/1 -> Camera_tl/1

== system W04_Town_cs/Controller ==
  Terminator : Terminator
  sfun_Controller : S-Function  FunctionName=sfun_Controller  Parameters=SParameter1, SParameter2, SParameter3, SParameter4, SParameter5, SParameter6, SParameter7, SParameter8, SParameter9, SParameter10, SampleTime  SFunctionDeploymentMode=off  EnableBusSupport=off  mask(Legacy Function){SFunctionSpec=void prescan_outputFcn(void** work1, PRESCAN_CONTROLLERDATA y1[1]), SParameter1=uint8([ExperimentFile 0]), SParameter2=uint8([ModelDepo 0]), SParameter3=uint8([ControllerOptions 0]), SParameter4=RTmode, SParameter5=PreScanExecutionMode, SParameter6=ControlMode, SParameter7=ControllerCount, SParameter8=ControllerIndex, SParameter9=uint8([SimulationMode 0]), SParameter10=uint8([TargetName 0]), SampleTime=TimeStep, ShowSpec=on}
      mask prompts: SParameter1 "P1:"; SParameter2 "P2:"; SParameter3 "P3:"; SParameter4 "P4:"; SParameter5 "P5:"; SParameter6 "P6:"; SParameter7 "P7:"; SParameter8 "P8:"; SParameter9 "P9:"; SParameter10 "P10:"; SampleTime "Sample time (-1 for inherited):"; ShowSpec "Display function specification"
      mask help:
      | This block allows you to call the legacy functions specified by the following Legacy Code Tool definition:
      | def.SFunctionName = 'sfun_Controller';
      | def.OutputFcnSpec = 'void prescan_outputFcn(void** work1, PRESCAN_CONTROLLERDATA y1[1])';
      | def.StartFcnSpec = 'void prescan_startFcn(void ** work1, uint8 p1[], uint8 p2[], uint8 p3[], double p4, double p5, double p6, double p7, double p8, uint8 p9[], uint8 p10[])';
      | def.TerminateFcnSpec = 'void prescan_terminateFcn(void** work1)';
      | def.HeaderFiles = {'prescan_controller_data.h', 'prescan_SFunLibrary.h', 'prescan_CreateLogHandler.h', 'prescan_CreateErrorHandler.h', 'prescan_modify.h', 'ModuleDLL.h'};
      | def.SourceFiles = {'prescan_MexLogHandler.c', 'prescan_SimStructErrorHandler.c', 'prescan_LogHandler.c', 'prescan_ErrorHandler.c', 'prescan_Modify.c'};
      | def.HostLibFiles = {'sensorinterfaced.lib'};
      | def.TargetLibFiles = {'sensorinterfaced.so'};
      | def.IncPaths = {'.', 'C:\projects\prescan\rt_vislibrary\vis\..\pimp\include\sensors\InterfaceRTW'};
      | def.SrcPaths = {'C:\projects\prescan\rt_vislibrary\vis\..\pimp\include\sensors\InterfaceRTW', 'C:\projects\prescan\rt_vislibrary\vis\..\pimp\include\sensors\InterfaceRTW\ccurrt'};
      | def.LibPaths = {'C:\\projects\\prescan\\vislibrary_build\lib'};
      | def.SampleTime = 'parameterized';
      mask Help: <p>This block was generated automatically by the Legacy Code Tool. For detailed help on this tool, call<a href="matlab:legacy_code('help')"> legacy_code('help')</a>.</p>
      mask Callback ShowSpec:
      | if strcmp(get_param(gcbh, 'ShowSpec'), 'on')
      |   set_param(gcbh, 'MaskDisplay', sprintf('fprintf(''%s'');', get_param(gcbh, 'SFunctionSpec')));
      | else
      |   set_param(gcbh, 'MaskDisplay', sprintf('fprintf(''%s'');', get_param(gcbh, 'FunctionName')));
      | end
      mask Display: fprintf('void prescan_outputFcn(void** work1, PRESCAN_CONTROLLERDATA y1[1])');
  wires:
  sfun_Controller/1 -> Terminator/1

== system W04_Town_cs/HumViewCamera ==
  Sensor : S-Function  FunctionName=sfun_Camera  Parameters=sensorID, dataWidth, dataHeight, channelsPerImage, numberOfImages, timestep  SFunctionDeploymentMode=off  EnableBusSupport=off  mask(PreScan Source Block: Camera Sensor){sensorID=16399, dataWidth=1080, dataHeight=5613, channelsPerImage=3, numberOfImages=1, timestep=1/20}
      mask prompts: sensorID "Sensor ID"; dataWidth "Data width"; dataHeight "Data Height"; channelsPerImage "Channels per image"; numberOfImages "Number of images"; timestep "MATLAB timestep:"
      mask help: The Camera Sensor provides a color or monochrome image.
      mask Help: eval('openHelp(457)')
      mask Display: image(imread('CameraSensor.png'))
  HumViewCamera : Outport  Tag=outport/Camera/CameraSensor  OutDataTypeStr=uint8  SampleTime=1/20
  wires:
  Sensor/1 -> HumViewCamera/1

== system W04_Town_cs/PointCloudSensor_1 ==
  Sensor : S-Function  FunctionName=sfun_PCS  Parameters=sensorID, dataWidth, dataHeight, numChannels, dataType, timestep  SFunctionDeploymentMode=off  EnableBusSupport=off  mask(PreScan Source Block: Point Cloud Sensor){sensorID=16393, dataWidth=16, dataHeight=900, numChannels=4, dataType=0, timestep=1/20}
      mask prompts: sensorID "Sensor ID"; dataWidth "Data Width"; dataHeight "Data Height"; numChannels "Channel Count"; dataType "Data Type"; timestep "MATLAB timestep:"
      mask help: The Point Cloud Sensor provides XYZ positions relative to the sensor
      mask Help: eval('openHelp(6400)')
      mask Display: image(imread('PointCloudSensorSL.png'))
  PointCloudSensor_1 : Outport  Tag=outport/PointCloudInport  OutDataTypeStr=single  SampleTime=1/20
  wires:
  Sensor/1 -> PointCloudSensor_1/1
